simulink model "EV_Simple"  (R2022b)
settings: Solver=FixedStepAuto  StartTime=0.0  StopTime=StopTime  RelTol=1e-3
values from neighbouring files (symbols this model uses):
  AccessoryLoad = 100    [EV_Simple_Mass_CdAf.m]    (also in EV_Simple_Params.m; matlab.mat = 600)
  airDensity = 1.293    [EV_Simple_Mass_CdAf.m]    (also in EV_Simple_Params.m; matlab.mat = 12.6)
  cdaf = CdAfRange(n)    [EV_Simple_Mass_CdAf.m]    (also in EV_Simple_Params.m = 0.21981)
  D_Driver = 0    [EV_Simple_Mass_CdAf.m]    (also in EV_Simple_Params.m; matlab.mat)
  energyCapacity = 2    [EV_Simple_Mass_CdAf.m]    (also in EV_Simple_Params.m; matlab.mat = 12.6)
  GR = Ndriven/Ndriving    (= 4)    [EV_Simple_Params.m]
  gravity = 9.81    [EV_Simple_Mass_CdAf.m]    (also in EV_Simple_Params.m; matlab.mat)
  I_Driver = 1    [EV_Simple_Mass_CdAf.m]    (also in EV_Simple_Params.m = 0.4; matlab.mat)
  initialSOC = 0.95    [EV_Simple_Mass_CdAf.m]    (also in EV_Simple_Params.m; matlab.mat)
  internalResistance = 0.05    [EV_Simple_Mass_CdAf.m]    (also in EV_Simple_Params.m; matlab.mat = 0.1)
  massVeh = massRange(m)    [EV_Simple_Mass_CdAf.m]    (also in EV_Simple_Params.m = 173; matlab.mat = 2000)
  maxBrakeForce = -400    [EV_Simple_Params.m]
  MotorC = 628.2974    [EV_Simple_Mass_CdAf.m]    (also in EV_Simple_Params.m; matlab.mat)
  MotorKc = 0.0452    [EV_Simple_Mass_CdAf.m]    (also in EV_Simple_Params.m; matlab.mat)
  MotorKi = 0.0167    [EV_Simple_Mass_CdAf.m]    (also in EV_Simple_Params.m; matlab.mat)
  MotorKw = 5.0664e-5    (= 5.0664e-05)    [EV_Simple_Mass_CdAf.m]    (also in EV_Simple_Params.m; matlab.mat)
  motorMaxPower = 2e3    (= 2000)    [EV_Simple_Params.m]
  motorMaxTorque = 15    [EV_Simple_Params.m]
  openCircuitVoltage = 52    [EV_Simple_Mass_CdAf.m]    (also in EV_Simple_Params.m; matlab.mat = 340)
  P_Driver = 250    [EV_Simple_Mass_CdAf.m]    (also in EV_Simple_Params.m = 225; matlab.mat)
  r_wheel = .254    (= 0.254)    [EV_Simple_Params.m]
  rollingResistCoeff = 0.01    [EV_Simple_Mass_CdAf.m]    (also in EV_Simple_Params.m; matlab.mat)
  Spinloss = 6    [EV_Simple_Mass_CdAf.m]    (also in EV_Simple_Params.m; matlab.mat)
  time_step = time(2)    [EV_Simple_Mass_CdAf.m]    (also in EV_Simple_Params.m; matlab.mat = 0.01)
undefined symbols (not defined in the file or in its folder): magnitude
libraries: simulink x3, slpidlib x1
settings Model: Creator=skylarlennon  LastModifiedBy=skylarlennon
settings DataIOCC: SaveFormat=Array  ReturnWorkspaceOutputs=off

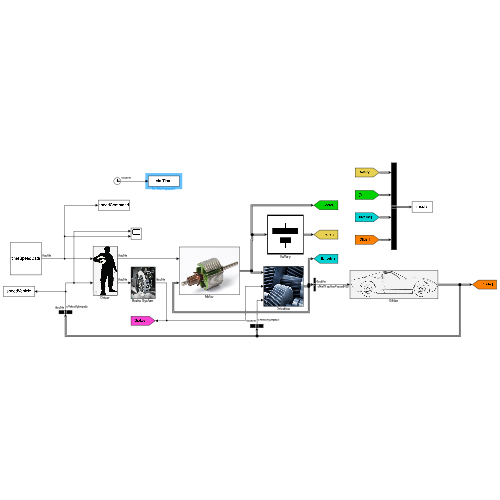
[thumbnail: Simulink's stored preview of the top-level diagram]
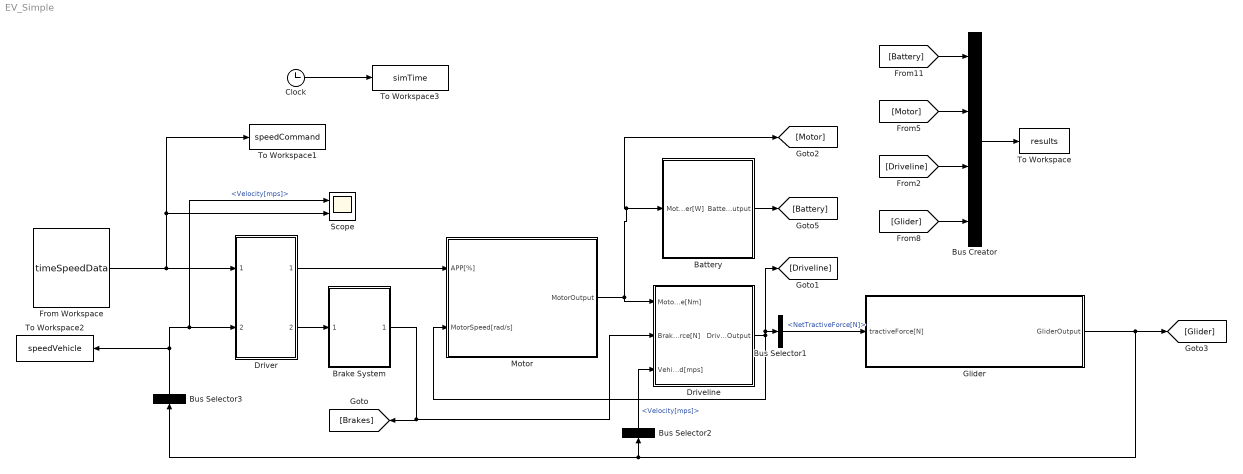
== system EV_Simple ==
  Battery : Subsystem
      mask Display: image('battery.jpg');
  Brake System : Subsystem
      mask Display: image('$imagefile'); % Use "Edit Image" on toolstrip to change.
  Bus Creator : BusCreator  Inputs=4
  Bus Selector1 : BusSelector  OutputSignals=NetTractiveForce[N]
  Bus Selector2 : BusSelector  OutputSignals=Velocity[mps]
  Bus Selector3 : BusSelector  OutputSignals=Velocity[mps]
  Clock : Clock
  Driveline : Subsystem
      mask Display: image('$imagefile'); % Use "Edit Image" on toolstrip to change.
  Driver : Subsystem  AncestorBlock=Driver_Glider_Library/Driver
      mask Display: image('$imagefile'); % Use "Edit Image" on toolstrip to change.
  From Workspace : FromWorkspace  VariableName=timeSpeedData  SampleTime=time_step
  Glider : Subsystem
      mask Display: image('$imagefile'); % Use "Edit Image" on toolstrip to change.
  Motor : Subsystem
      mask Display: image('$imagefile'); % Use "Edit Image" on toolstrip to change.
  Scope : Scope  NumInputPorts=2
  To Workspace : ToWorkspace  VariableName=results  SampleTime=-1
  To Workspace1 : ToWorkspace  VariableName=speedCommand  SampleTime=-1
  To Workspace2 : ToWorkspace  VariableName=speedVehicle  SampleTime=-1
  To Workspace3 : ToWorkspace  VariableName=simTime  SampleTime=-1
  wires:
  Driver/2(BPP[%]) -> Brake System/1(BPP[%])
  Driver/1(APP[%]) -> Motor/1(APP[%])
  [Glider] -> Bus Creator/4
  [Motor] -> Bus Creator/2
  Bus Creator/1 -> To Workspace/1
  [Driveline] -> Bus Creator/3
  [Battery] -> Bus Creator/1
  Motor/1(MotorOutput) -> Driveline/1(MotorTorque[Nm]), [Motor], Battery/1(MotorPower[W])
  Battery/1(BatteryOutput) -> [Battery]
  Brake System/1(BrakeOutput) -> Driveline/2(BrakeForce[N]), [Brakes]
  Bus Selector1/1 -> Glider/1(tractiveForce[N])  "<NetTractiveForce[N]>"
  Driveline/1(DrivelineOutput) -> Bus Selector1/1, [Driveline], Motor/2(MotorSpeed[rad/s])
  Glider/1(GliderOutput) -> [Glider], Bus Selector2/1, Bus Selector3/1
  Bus Selector2/1 -> Driveline/3(VehicleSpeed[mps])  "<Velocity[mps]>"
  Bus Selector3/1 -> Scope/1, Driver/2(VehicleSpeed[mph]), To Workspace2/1  "<Velocity[mps]>"
  From Workspace/1 -> To Workspace1/1, Scope/2, Driver/1(VehicleSpeedRef)
  Clock/1 -> To Workspace3/1

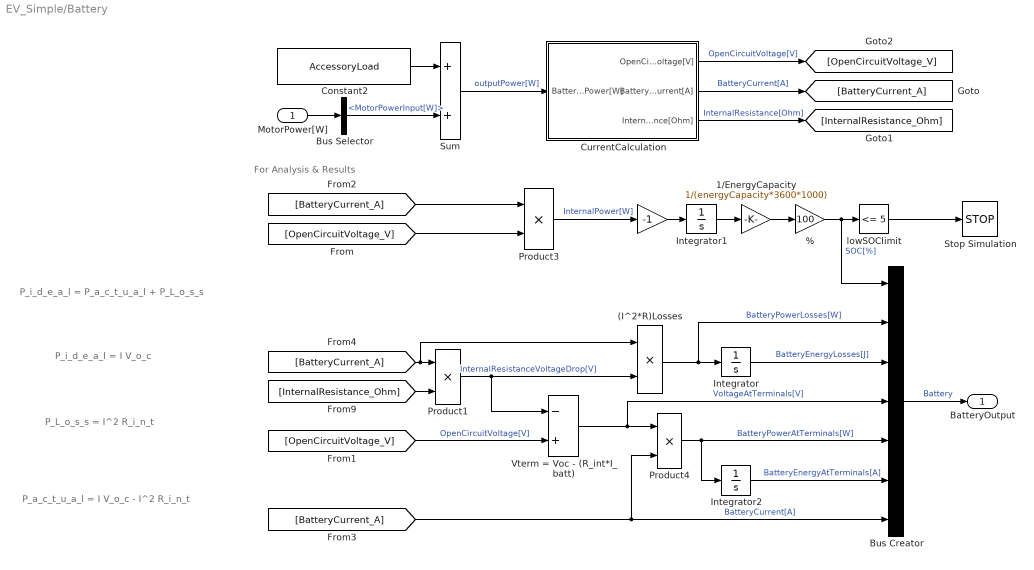
== system EV_Simple/Battery ==
  note: For Analysis & Results
  note: P_i_d_e_a_l = I V_o_c
  note: P_i_d_e_a_l = P_a_c_t_u_a_l + P_L_o_s_s
  note: P_L_o_s_s = I^2 R_i_n_t
  note: P_a_c_t_u_a_l = I V_o_c - I^2 R_i_n_t
  MotorPower[W] : Inport
  " " : Gain  Gain=-1
  % : Gain  Gain=100
  (I^2*R)Losses : Product  RndMeth=Zero
  1/EnergyCapacity : Gain  Gain=1/(energyCapacity*3600*1000)
  Bus Creator : BusCreator  Inputs=7
  Bus Selector : BusSelector  OutputSignals=MotorPowerInput[W]
  Constant2 : Constant  Value=AccessoryLoad
  CurrentCalculation : Subsystem
  Integrator : Integrator  ZeroCross=off
  Integrator1 : Integrator  InitialCondition=energyCapacity*3600*1000*initialSOC  ZeroCross=off
  Integrator2 : Integrator
  Product1 : Product  RndMeth=Zero
  Product3 : Product  RndMeth=Zero
  Product4 : Product  RndMeth=Zero
  Stop Simulation : Stop
  Sum : Sum
  Vterm = Voc - (R_int*I_batt) : Sum  Inputs=-+
  lowSOClimit : simulink/Logic and Bit Operations/Compare To Constant  relop=<=  const=5  OutDataTypeStr=boolean
  BatteryOutput : Outport  VectorParamsAs1DForOutWhenUnconnected=off
  wires:
  Product1/1 -> (I^2*R)Losses/2, Vterm = Voc - (R_int*I_batt)/1  "InternalResistanceVoltageDrop[V]"
  (I^2*R)Losses/1 -> Bus Creator/2, Integrator/1  "BatteryPowerLosses[W]"
  Integrator/1 -> Bus Creator/3  "BatteryEnergyLosses[J]"
  Product3/1 -> " "/1  "InternalPower[W]"
  Integrator1/1 -> 1/EnergyCapacity/1
  Constant2/1 -> Sum/1
  Bus Creator/1 -> BatteryOutput/1  "Battery"
  1/EnergyCapacity/1 -> %/1
  MotorPower[W]/1 -> Bus Selector/1
  Sum/1 -> CurrentCalculation/1(BatteryPower[W])  "outputPower[W]"
  " "/1 -> Integrator1/1
  Bus Selector/1 -> Sum/2  "<MotorPowerInput[W]>"
  [OpenCircuitVoltage_V] -> Product3/2
  CurrentCalculation/1(OpenCircuitVoltage[V]) -> [OpenCircuitVoltage_V]  "OpenCircuitVoltage[V]"
  [OpenCircuitVoltage_V] -> Vterm = Voc - (R_int*I_batt)/2  "OpenCircuitVoltage[V]"
  [BatteryCurrent_A] -> Product3/1
  [BatteryCurrent_A] -> Bus Creator/7, Product4/2  "BatteryCurrent[A]"
  [BatteryCurrent_A] -> (I^2*R)Losses/1, Product1/1
  Vterm = Voc - (R_int*I_batt)/1 -> Bus Creator/4, Product4/1  "VoltageAtTerminals[V]"
  CurrentCalculation/2(BatteryCurrent[A]) -> [BatteryCurrent_A]  "BatteryCurrent[A]"
  CurrentCalculation/3(InternalResistance[Ohm]) -> [InternalResistance_Ohm]  "InternalResistance[Ohm]"
  [InternalResistance_Ohm] -> Product1/2
  Product4/1 -> Bus Creator/5, Integrator2/1  "BatteryPowerAtTerminals[W]"
  Integrator2/1 -> Bus Creator/6  "BatteryEnergyAtTerminals[A]"
  %/1 -> lowSOClimit/1, Bus Creator/1  "SOC[%]"
  lowSOClimit/1 -> Stop Simulation/1

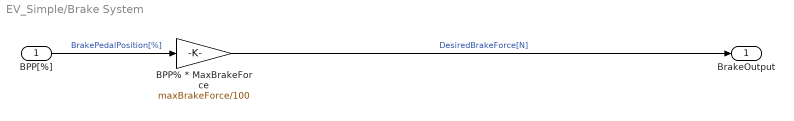
== system EV_Simple/Brake System ==
  BPP[%] : Inport
  BPP% * MaxBrakeForce : Gain  Gain=maxBrakeForce/100
  BrakeOutput : Outport  VectorParamsAs1DForOutWhenUnconnected=off
  wires:
  BPP[%]/1 -> BPP% * MaxBrakeForce/1  "BrakePedalPosition[%]"
  BPP% * MaxBrakeForce/1 -> BrakeOutput/1  "DesiredBrakeForce[N]"

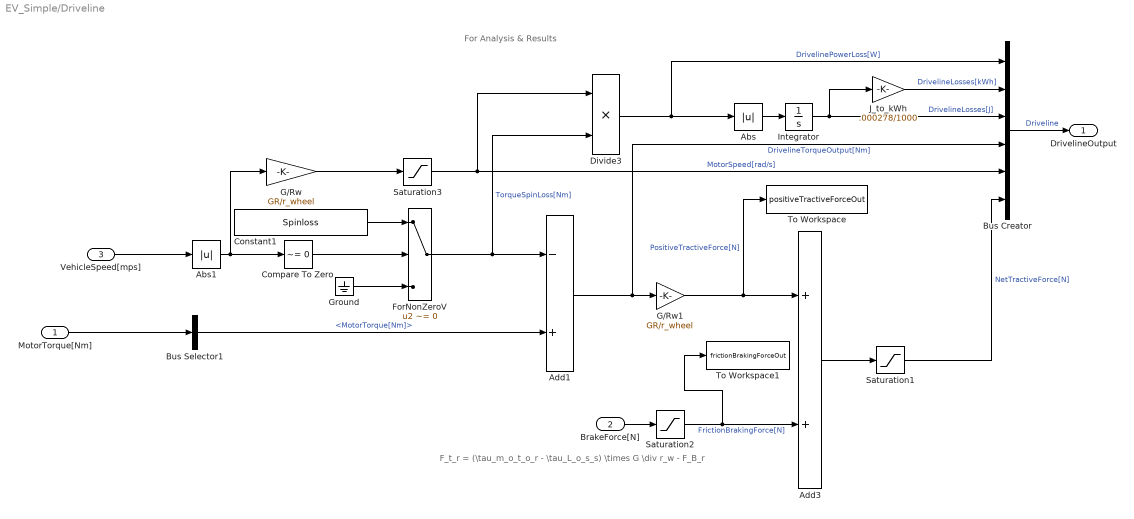
== system EV_Simple/Driveline ==
  note: For Analysis & Results
  note: F_t_r = (\tau_m_o_t_o_r - \tau_L_o_s_s) \times G \div r_w - F_B_r
  MotorTorque[Nm] : Inport
  BrakeForce[N] : Inport  Port=2
  VehicleSpeed[mps] : Inport  Port=3
  Abs : Abs  ZeroCross=off  SaturateOnIntegerOverflow=off
  Abs1 : Abs  ZeroCross=off  SaturateOnIntegerOverflow=off
  Add1 : Sum  Inputs=-+
  Add3 : Sum
  Bus Creator : BusCreator  Inputs=6
  Bus Selector1 : BusSelector  OutputSignals=MotorTorque[Nm]
  Compare To Zero : simulink/Logic and Bit Operations/Compare To Zero  relop=~=  OutDataTypeStr=boolean
  Constant1 : Constant  Value=Spinloss
  Divide3 : Product  Inputs=**
  ForNonZeroV : Switch  Criteria=u2 ~= 0  ZeroCross=off  SaturateOnIntegerOverflow=off  InputSameDT=off
  G/Rw : Gain  Gain=GR/r_wheel
  G/Rw1 : Gain  Gain=GR/r_wheel
  Ground : Ground
  Integrator : Integrator  ZeroCross=off
  J_to_kWh : Gain  Gain=.000278/1000
  Saturation1 : Saturate  UpperLimit=5000  LowerLimit=-10000  ZeroCross=off
  Saturation2 : Saturate  UpperLimit=0  LowerLimit=-10000  ZeroCross=off
  Saturation3 : Saturate  UpperLimit=inf  LowerLimit=0.00001  ZeroCross=off
  To Workspace : ToWorkspace  VariableName=positiveTractiveForceOut  SampleTime=-1
  To Workspace1 : ToWorkspace  VariableName=frictionBrakingForceOut  SampleTime=-1
  DrivelineOutput : Outport  VectorParamsAs1DForOutWhenUnconnected=off
  wires:
  G/Rw1/1 -> To Workspace/1, Add3/1  "PositiveTractiveForce[N]"
  Add3/1 -> Saturation1/1
  Abs/1 -> Integrator/1
  Saturation2/1 -> To Workspace1/1, Add3/2  "FrictionBrakingForce[N]"
  MotorTorque[Nm]/1 -> Bus Selector1/1
  G/Rw/1 -> Saturation3/1
  ForNonZeroV/1 -> Divide3/2, Add1/1  "TorqueSpinLoss[Nm]"
  Add1/1 -> G/Rw1/1, Bus Creator/4  "DrivelineTorqueOutput[Nm]"
  Saturation3/1 -> Divide3/1, Bus Creator/5  "MotorSpeed[rad/s]"
  Divide3/1 -> Bus Creator/1, Abs/1  "DrivelinePowerLoss[W]"
  Saturation1/1 -> Bus Creator/6  "NetTractiveForce[N]"
  Abs1/1 -> Compare To Zero/1, G/Rw/1
  BrakeForce[N]/1 -> Saturation2/1
  J_to_kWh/1 -> Bus Creator/2  "DrivelineLosses[kWh]"
  Ground/1 -> ForNonZeroV/3
  Constant1/1 -> ForNonZeroV/1
  Bus Creator/1 -> DrivelineOutput/1  "Driveline"
  Integrator/1 -> J_to_kWh/1, Bus Creator/3  "DrivelineLosses[J]"
  Bus Selector1/1 -> Add1/2  "<MotorTorque[Nm]>"
  Compare To Zero/1 -> ForNonZeroV/2
  VehicleSpeed[mps]/1 -> Abs1/1

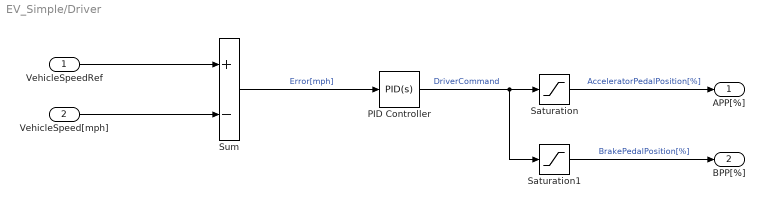
== system EV_Simple/Driver ==
  VehicleSpeedRef : Inport
  VehicleSpeed[mph] : Inport  Port=2
  PID Controller : slpidlib/PID Controller  Controller=PID  Form=Parallel  TimeDomain=Continuous-time  UseExternalTs=off  SampleTime=-1  IntegratorMethod=Forward Euler  FilterMethod=Forward Euler  ControllerParametersSource=internal  P=P_Driver  I=I_Driver  UseKiTs=off  D=D_Driver  N=100  UseFilter=on  TunerSelectOption=Transfer Function Based (PID Tuner App)  InitialConditionSource=internal  InitialConditionForIntegrator=0  InitialConditionForFilter=0  DifferentiatorICPrevScaledInput=0  ExternalReset=none  TrackingMode=off  Kt=1  LimitOutput=off  SatLimitsSource=internal  UpperSaturationLimit=inf  LowerSaturationLimit=-inf  LinearizeAsGain=on  AntiWindupMode=none  Kb=1  LimitIntegrator=off  UpperIntegratorSaturationLimit=inf  LowerIntegratorSaturationLimit=-inf  POutMin=[]  POutMax=[]  IOutMin=[]  IOutMax=[]  DOutMin=[]  DOutMax=[]  NOutMin=[]  NOutMax=[]  SumOutMin=[]  SumOutMax=[]  SaturationOutMin=[]  SaturationOutMax=[]  PParamMin=[]  PParamMax=[]  IParamMin=[]  IParamMax=[]  DParamMin=[]  DParamMax=[]  NParamMin=[]  NParamMax=[]  KbParamMin=[]  KbParamMax=[]  KtParamMin=[]  KtParamMax=[]  KbOutMin=[]  KbOutMax=[]  KtOutMin=[]  KtOutMax=[]  IntegratorOutMin=[]  IntegratorOutMax=[]  FilterOutMin=[]  FilterOutMax=[]  SumI1OutMin=[]  SumI1OutMax=[]  SumI2OutMin=[]  SumI2OutMax=[]  SumI3OutMin=[]  SumI3OutMax=[]  SumI4OutMin=[]  SumI4OutMax=[]  SumDOutMin=[]  SumDOutMax=[]  DifferentiatorOutMin=[]  DifferentiatorOutMax=[]  FilterDiffOutCoefMin=[]  FilterDiffOutCoefMax=[]  ReciprocalOutMin=[]  ReciprocalOutMax=[]  SumDenOutMin=[]  SumDenOutMax=[]  SumNumOutMin=[]  SumNumOutMax=[]  DivideOutMin=[]  DivideOutMax=[]  UdiffTsProdOutMin=[]  UdiffTsProdOutMax=[]  NTsProdOutMin=[]  NTsProdOutMax=[]  UintegralTsProdOutMin=[]  UintegralTsProdOutMax=[]  UngainTsProdOutMin=[]  UngainTsProdOutMax=[]  ClampingZeroOutDataTypeStr=Inherit: Inherit via back propagation  ClampingZeroOutMin=[]  ClampingZeroOutMax=[]  FilterDenConstantOutDataTypeStr=Inherit: Inherit via back propagation  FilterDenConstantOutMin=[]  FilterDenConstantOutMax=[]  PCopyOutDataTypeStr=Inherit: Inherit via back propagation  PCopyOutMin=[]  PCopyOutMax=[]  NCopyOutDataTypeStr=Inherit: Inherit via back propagation  NCopyOutMin=[]  NCopyOutMax=[]  IntegratorContinuousStateAttributes=''  IntegratorStateMustResolveToSignalObject=off  IntegratorRTWStateStorageClass=Auto  FilterContinuousStateAttributes=''  FilterStateMustResolveToSignalObject=off  FilterRTWStateStorageClass=Auto  ParallelPVariant=InternalParameters  IdealPVariant=Disabled  IVariant=InternalParameters  DVariant=InternalParameters  IntegratorVariant=Continuous  SatVariant=Disabled  AWVariant=Passthrough  PCopyVariant=Disabled  TRVariant=Disabled  FdbkBlocksVariant=Forward  IdealPFdbkVariant=Disabled  SatFdbkVariant=Disabled  DerivativeFilterVariant=ContFilter  NVariant=InternalParameters  NCopyVariant=Disabled  FilterICVariant=InternalICsFilter  IntegratorICVariant=InternalICs  ExternalResetVariant=Disabled  TRSumVariant=Passthrough  SumFdbkVariant=Disabled  SumVariant=Sum_PID  TsampFilterVariant=InternalTs  TsampNgainVariant=Passthrough  TsampIntegralVariant=Passthrough  ExternalSaturationOutDataTypeStr=Inherit: Same as second input
  Saturation : Saturate  UpperLimit=100  LowerLimit=0  ZeroCross=off
  Saturation1 : Saturate  UpperLimit=0  LowerLimit=-100  ZeroCross=off
  Sum : Sum  Inputs=+-
  APP[%] : Outport  VectorParamsAs1DForOutWhenUnconnected=off
  BPP[%] : Outport  Port=2  VectorParamsAs1DForOutWhenUnconnected=off
  wires:
  VehicleSpeed[mph]/1 -> Sum/2
  Sum/1 -> PID Controller/1  "Error[mph]"
  Saturation1/1 -> BPP[%]/1  "BrakePedalPosition[%]"
  PID Controller/1 -> Saturation/1, Saturation1/1  "DriverCommand"
  Saturation/1 -> APP[%]/1  "AcceleratorPedalPosition[%]"
  VehicleSpeedRef/1 -> Sum/1

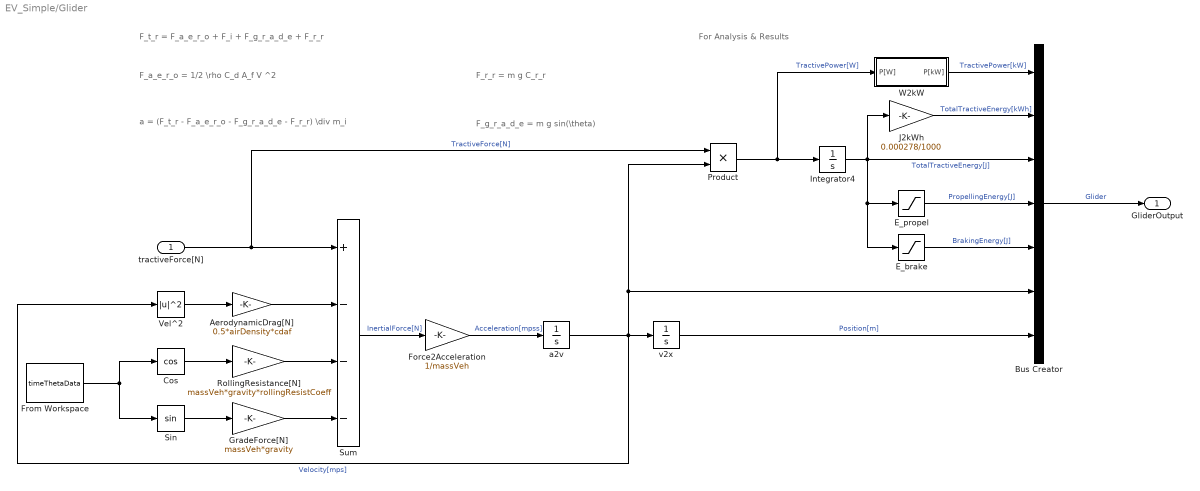
== system EV_Simple/Glider ==
  note: F_t_r = F_a_e_r_o + F_i + F_g_r_a_d_e + F_r_r
  note: a = (F_t_r - F_a_e_r_o - F_g_r_a_d_e - F_r_r) \div m_i
  note: F_r_r = m g C_r_r
  note: For Analysis & Results
  note: F_a_e_r_o = 1/2 \rho C_d A_f V ^2
  note: F_g_r_a_d_e = m g sin(\theta)
  tractiveForce[N] : Inport
  AerodynamicDrag[N] : Gain  Gain=0.5*airDensity*cdaf
      settings: AttributesFormatString=%<Gain>
  Bus Creator : BusCreator  Inputs=7
  Cos : Trigonometry  Operator=cos
  E_brake : Saturate  UpperLimit=0  LowerLimit=-inf
  E_propel : Saturate  UpperLimit=inf  LowerLimit=0
  Force2Acceleration : Gain  Gain=1/massVeh
      settings: AttributesFormatString=%<Gain>
  From Workspace : FromWorkspace  VariableName=timeThetaData
  GradeForce[N] : Gain  Gain=massVeh*gravity
  Integrator4 : Integrator
  J2kWh : Gain  Gain=0.000278/1000
  Product : Product
  RollingResistance[N] : Gain  Gain=massVeh*gravity*rollingResistCoeff
  Sin : Trigonometry
  Sum : Sum  Inputs=+---
  Vel^2 : Math  Operator=magnitude^2  SignedPower=on
  W2kW : Subsystem
  a2v : Integrator
  v2x : Integrator
  GliderOutput : Outport  VectorParamsAs1DForOutWhenUnconnected=off
  wires:
  J2kWh/1 -> Bus Creator/2  "TotalTractiveEnergy[kWh]"
  Sum/1 -> Force2Acceleration/1  "InertialForce[N]"
  E_propel/1 -> Bus Creator/4  "PropellingEnergy[J]"
  W2kW/1(P[kW]) -> Bus Creator/1  "TractivePower[kW]"
  Vel^2/1 -> AerodynamicDrag[N]/1
  Integrator4/1 -> J2kWh/1, Bus Creator/3, E_brake/1, E_propel/1  "TotalTractiveEnergy[J]"
  Force2Acceleration/1 -> a2v/1  "Acceleration[mpss]"
  E_brake/1 -> Bus Creator/5  "BrakingEnergy[J]"
  RollingResistance[N]/1 -> Sum/3
  GradeForce[N]/1 -> Sum/4
  AerodynamicDrag[N]/1 -> Sum/2
  v2x/1 -> Bus Creator/7  "Position[m]"
  a2v/1 -> v2x/1, Vel^2/1, Bus Creator/6, Product/2  "Velocity[mps]"
  tractiveForce[N]/1 -> Product/1, Sum/1  "TractiveForce[N]"
  Product/1 -> W2kW/1(P[W]), Integrator4/1  "TractivePower[W]"
  Bus Creator/1 -> GliderOutput/1  "Glider"
  From Workspace/1 -> Sin/1, Cos/1
  Cos/1 -> RollingResistance[N]/1
  Sin/1 -> GradeForce[N]/1

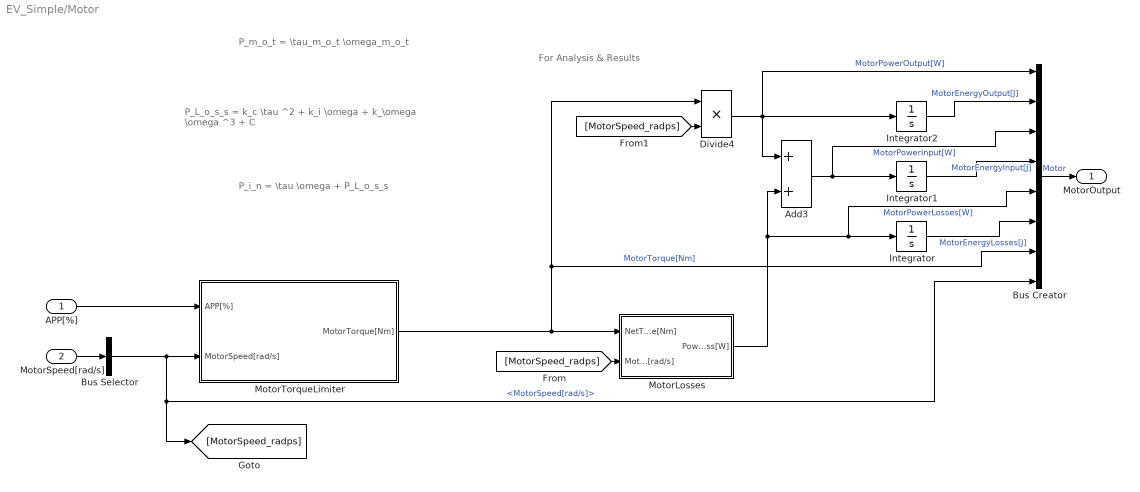
== system EV_Simple/Motor ==
  note: P_i_n = \tau \omega + P_L_o_s_s
  note: For Analysis & Results
  note: P_L_o_s_s = k_c \tau ^2 + k_i \omega + k_\omega \omega ^3 + C
  note: P_m_o_t = \tau_m_o_t \omega_m_o_t
  APP[%] : Inport
  MotorSpeed[rad/s] : Inport  Port=2
  Add3 : Sum
  Bus Creator : BusCreator  Inputs=8
  Bus Selector : BusSelector  OutputSignals=MotorSpeed[rad/s]
  Divide4 : Product  Inputs=**
  Integrator : Integrator  ZeroCross=off
  Integrator1 : Integrator  ZeroCross=off
  Integrator2 : Integrator  ZeroCross=off
  MotorLosses : Subsystem
  MotorTorqueLimiter : Subsystem
  MotorOutput : Outport  VectorParamsAs1DForOutWhenUnconnected=off
  wires:
  Add3/1 -> Bus Creator/3, Integrator1/1  "MotorPowerInput[W]"
  Divide4/1 -> Bus Creator/1, Add3/1, Integrator2/1  "MotorPowerOutput[W]"
  [MotorSpeed_radps] -> Divide4/2
  Integrator1/1 -> Bus Creator/4  "MotorEnergyInput[J]"
  Integrator2/1 -> Bus Creator/2  "MotorEnergyOutput[J]"
  MotorTorqueLimiter/1(MotorTorque[Nm]) -> Divide4/1, Bus Creator/7, MotorLosses/1(NetTorque[Nm])  "MotorTorque[Nm]"
  APP[%]/1 -> MotorTorqueLimiter/1(APP[%])
  MotorLosses/1(PowerLoss[W]) -> Bus Creator/5, Integrator/1, Add3/2  "MotorPowerLosses[W]"
  [MotorSpeed_radps] -> MotorLosses/2(MotorSpeed[rad/s])
  Bus Creator/1 -> MotorOutput/1  "Motor"
  Integrator/1 -> Bus Creator/6  "MotorEnergyLosses[J]"
  MotorSpeed[rad/s]/1 -> Bus Selector/1
  Bus Selector/1 -> MotorTorqueLimiter/2(MotorSpeed[rad/s]), Bus Creator/8, [MotorSpeed_radps]  "<MotorSpeed[rad/s]>"

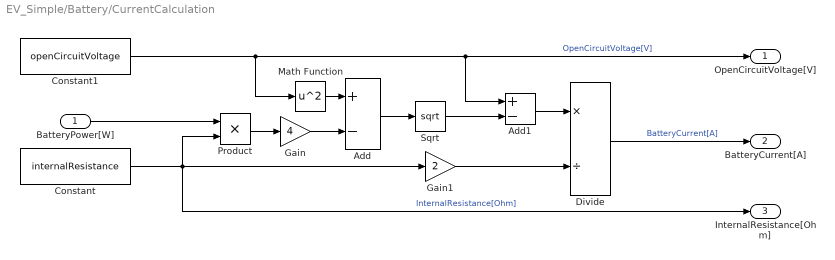
== system EV_Simple/Battery/CurrentCalculation ==
  BatteryPower[W] : Inport
  Add : Sum  Inputs=+-
  Add1 : Sum  Inputs=+-
  Constant : Constant  Value=internalResistance
  Constant1 : Constant  Value=openCircuitVoltage
  Divide : Product  Inputs=*/
  Gain : Gain  Gain=4
  Gain1 : Gain  Gain=2
  Math Function : Math  Operator=square  SignedPower=on
  Product : Product  RndMeth=Zero
  Sqrt : Sqrt
  OpenCircuitVoltage[V] : Outport  VectorParamsAs1DForOutWhenUnconnected=off
  BatteryCurrent[A] : Outport  Port=2  VectorParamsAs1DForOutWhenUnconnected=off
  InternalResistance[Ohm] : Outport  Port=3  VectorParamsAs1DForOutWhenUnconnected=off
  wires:
  BatteryPower[W]/1 -> Product/1
  Constant/1 -> InternalResistance[Ohm]/1, Gain1/1, Product/2  "InternalResistance[Ohm]"
  Product/1 -> Gain/1
  Constant1/1 -> Math Function/1, OpenCircuitVoltage[V]/1, Add1/1  "OpenCircuitVoltage[V]"
  Math Function/1 -> Add/1
  Gain/1 -> Add/2
  Sqrt/1 -> Add1/2
  Add/1 -> Sqrt/1
  Add1/1 -> Divide/1
  Gain1/1 -> Divide/2
  Divide/1 -> BatteryCurrent[A]/1  "BatteryCurrent[A]"

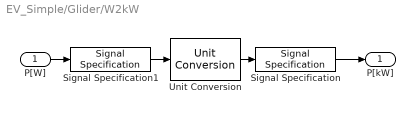
== system EV_Simple/Glider/W2kW ==
  P[W] : Inport
  Signal Specification : SignalSpecification  Unit=kW
  Signal Specification1 : SignalSpecification  Unit=W
  Unit Conversion : UnitConversion
  P[kW] : Outport  VectorParamsAs1DForOutWhenUnconnected=off
  wires:
  Signal Specification/1 -> P[kW]/1
  Signal Specification1/1 -> Unit Conversion/1
  Unit Conversion/1 -> Signal Specification/1
  P[W]/1 -> Signal Specification1/1

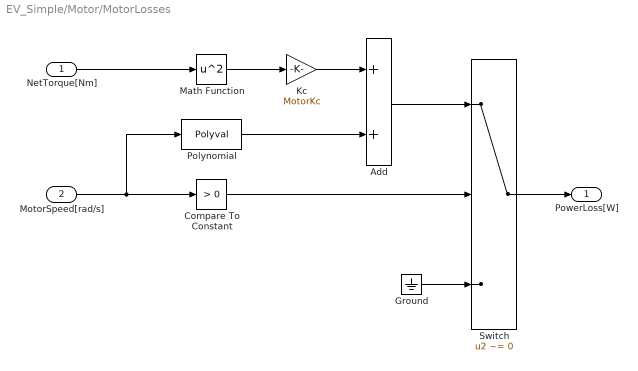
== system EV_Simple/Motor/MotorLosses ==
  NetTorque[Nm] : Inport
  MotorSpeed[rad/s] : Inport  Port=2
  Add : Sum
  Compare To Constant : simulink/Logic and Bit Operations/Compare To Constant  relop=>  const=0  OutDataTypeStr=boolean
  Ground : Ground
  Kc : Gain  Gain=MotorKc
  Math Function : Math  Operator=square  SignedPower=on
  Polynomial : Polyval  Coefs=[MotorKw , 0 ,MotorKi, MotorC]
  Switch : Switch  Criteria=u2 ~= 0  ZeroCross=off  SaturateOnIntegerOverflow=off  InputSameDT=off
  PowerLoss[W] : Outport  VectorParamsAs1DForOutWhenUnconnected=off
  wires:
  NetTorque[Nm]/1 -> Math Function/1
  Math Function/1 -> Kc/1
  Kc/1 -> Add/1
  MotorSpeed[rad/s]/1 -> Polynomial/1, Compare To Constant/1
  Ground/1 -> Switch/3
  Switch/1 -> PowerLoss[W]/1
  Polynomial/1 -> Add/2
  Add/1 -> Switch/1
  Compare To Constant/1 -> Switch/2

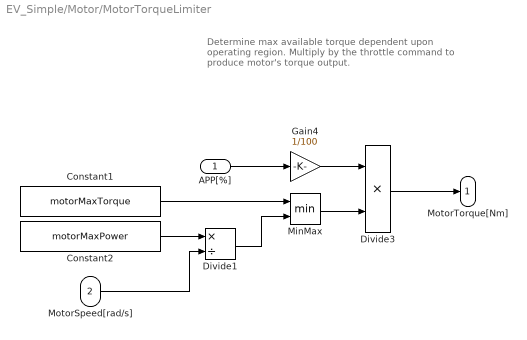
== system EV_Simple/Motor/MotorTorqueLimiter ==
  note: Determine max available torque dependent upon
      | operating region. Multiply by the throttle command
      | to produce motor's torque output.
  APP[%] : Inport
  MotorSpeed[rad/s] : Inport  Port=2
  Constant1 : Constant  Value=motorMaxTorque
  Constant2 : Constant  Value=motorMaxPower
  Divide1 : Product  Inputs=*/
  Divide3 : Product  Inputs=**
  Gain4 : Gain  Gain=1/100
  MinMax : MinMax  Inputs=2
  MotorTorque[Nm] : Outport  VectorParamsAs1DForOutWhenUnconnected=off
  wires:
  Constant1/1 -> MinMax/1
  MinMax/1 -> Divide3/2
  Gain4/1 -> Divide3/1
  APP[%]/1 -> Gain4/1
  Divide3/1 -> MotorTorque[Nm]/1
  Constant2/1 -> Divide1/1
  Divide1/1 -> MinMax/2
  MotorSpeed[rad/s]/1 -> Divide1/2
